simulink model "contorl_plc"  (R2013a)
settings: Solver=ode45  StartTime=0.0  StopTime=inf  RelTol=1e-3
undefined symbols (not defined in the file or in its folder): Bomba1, Bomba2, Opc_Teste, ref1, ref2, Tanq1, Tanq2, Tanq3, Tanq4, Test_Tags
libraries: opclib x3
settings Model: Creator=Administrator  LastModifiedBy=Administrator

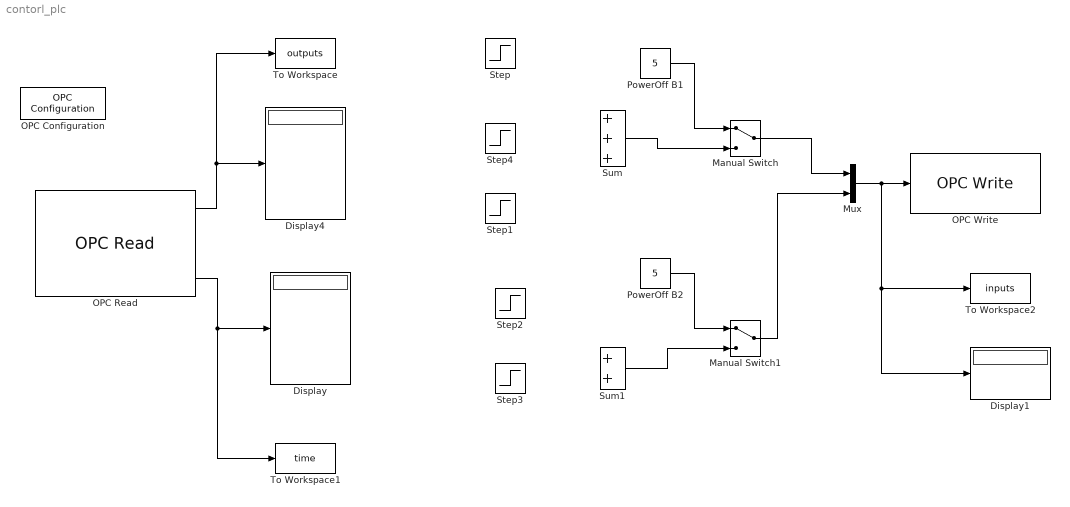
== system contorl_plc ==
  Display : Display
  Display1 : Display
  Display4 : Display
  Manual Switch : ManualSwitch
  Manual Switch1 : ManualSwitch
  Mux : Mux  Inputs=2
  OPC Configuration : opclib/OPC Configuration  opcServers=localhost/RSLinx OPC Server/10  errMissingItems=Error  errReadWrite=Warn  errShutdown=Error  errRTViolation=Warn  rtEnable=on  speedup=1  showLatency=off  beingUsed=on
  OPC Read : opclib/OPC Read  serverHost=localhost  serverID=RSLinx OPC Server  itemIDs=[Opc_Teste]Tanq4, [Opc_Teste]Tanq3, [Opc_Teste]Tanq2, [Opc_Teste]Tanq1, [Test_Tags]Bomba1, [Test_Tags]Bomba2  readMode=Synchronous (cache)  dataType=double  updateRate=0.2  showQual=on  showTS=on  tsMode=Seconds since start
  OPC Write : opclib/OPC Write  serverHost=localhost  serverID=RSLinx OPC Server  itemIDs=[Test_Tags]ref1, [Test_Tags]ref2  writeMode=Synchronous  updateRate=0.2
  PowerOff B1 : Constant  Value=5
  PowerOff B2 : Constant  Value=5
  Step : Step  Time=1500  Before=42  After=45
  Step1 : Step  Time=6000  After=-42
  Step2 : Step  Time=3000  Before=42  After=45
  Step3 : Step  Time=6000  After=-45
  Step4 : Step  Time=4500  After=-3
  Sum : Sum  Inputs=+++
  Sum1 : Sum
  To Workspace : ToWorkspace  VariableName=outputs  SampleTime=-1  SaveFormat=Timeseries
  To Workspace1 : ToWorkspace  VariableName=time  SampleTime=-1  SaveFormat=Timeseries
  To Workspace2 : ToWorkspace  VariableName=inputs  SampleTime=-1  SaveFormat=Timeseries
  wires:
  OPC Read/3 -> To Workspace1/1, Display/1
  OPC Read/1 -> To Workspace/1, Display4/1
  PowerOff B1/1 -> Manual Switch/1
  PowerOff B2/1 -> Manual Switch1/1
  Sum1/1 -> Manual Switch1/2
  Manual Switch/1 -> Mux/1
  Manual Switch1/1 -> Mux/2
  Mux/1 -> Display1/1, To Workspace2/1, OPC Write/1
  Sum/1 -> Manual Switch/2
